simulink model "untitled2"  (R2020b)
settings: Solver=VariableStepAuto  StartTime=0.0  StopTime=100  MaxStep=0.1  RelTol=1e-3
model workspace (MAT data in the model file):
  B = 50
  K = 50
  M1 = 100
settings Model: DataDictionary=untitled.sldd  OrderedModelArguments=off  Creator=user  LastModifiedBy=user
settings DataIOCC: ExternalInput=[t, road]  LoadExternalInput=on

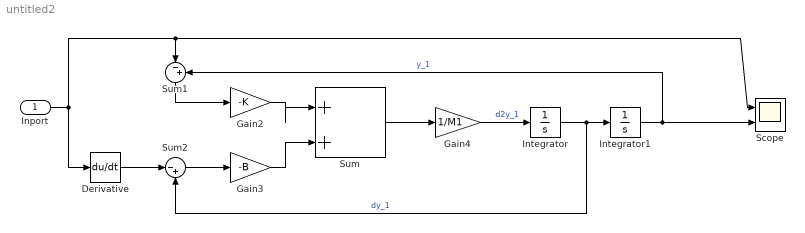
== system untitled2 ==
  Inport : Inport
  Derivative : Derivative
  Gain2 : Gain  Gain=-K
  Gain3 : Gain  Gain=-B
  Gain4 : Gain  Gain=1/M1
  Integrator : Integrator
  Integrator1 : Integrator
  Scope : Scope  NumInputPorts=2
  Sum : Sum  Inputs=|++
  Sum1 : Sum  Inputs=|-+
  Sum2 : Sum  Inputs=|-+
  wires:
  Integrator/1 -> Sum2/2, Integrator1/1  "dy_1"
  Sum/1 -> Gain4/1
  Gain4/1 -> Integrator/1  "d2y_1"
  Sum1/1 -> Gain2/1
  Sum2/1 -> Gain3/1
  Integrator1/1 -> Sum1/2, Scope/2  "y_1"
  Gain3/1 -> Sum/2
  Gain2/1 -> Sum/1
  Derivative/1 -> Sum2/1
  Inport/1 -> Scope/1, Sum1/1, Derivative/1
